simulink model "MPCtest1_real_44_double_lane_change"  (Simulink 8.7)
(part 2 of 4)

      | 6.247432626
      | 6.250432626
      | 6.253432626
      | 6.256432626
      | 6.259432626
      | 6.262432626
      | 6.265432626
      | 6.268432626
      | 6.271432626
      | 6.274432626
      | 6.277432626
      | 6.280432626
      | 6.283432626
      | 6.286432626
      | 6.289432626
      | 6.292432626
      | 6.295432626
      | 6.298432626
      | 6.301432626
      | 6.304432626
      | 6.307432626
      | 6.310432626
      | 6.313432626
      | 6.316432626
      | 6.319432626
      | ]*4
      | [0
      | 0
      | 0
      | 0
      | 0
      | 0
      | 0
      | 0
      | 0
      | 0
      | 0
      | 0
      | 0
      | 0
      | 0
      | 0
      | 0
      | 0
      | 0
      | 0
      | 0
      | 0
      | 0
      | 0
      | 0
      | 0
      | 0
      | 0
      | 0
      | 0
      | 0
      | 0
      | 0
      | 0
      | 0
      | 0
      | 0
      | 0
      | 0
      | 0
      | 0
      | 0
      | 0
      | 0
      | 0
      | 0
      | 0
      | 0
      | 0
      | 0
      | 0
      | 0
      | 0
      | 0
      | 0
      | 0
      | 0
      | 0
      | 0
      | 0
      | 0
      | 0
      | 0
      | 0
      | 0
      | 0
      | 0
      | 0
      | 0
      | 0
      | 0
      | 0
      | 0
      | 0
      | 0
      | 0
      | 0
      | 0
      | 0
      | 0
      | 0
      | 0
      | 0
      | 0
      | 0
      | 0
      | 0
      | 0
      | 0
      | 0
      | 0
      | 0
      | 0
      | 0
      | 0
      | 0
      | 0
      | 0
      | 0
      | 0
      | 0
      | 0
      | 0
      | 0
      | 0
      | 0
      | 0
      | 0
      | 0
      | 0
      | 0
      | 0
      | 0
      | 0
      | 0
      | 0
      | 0
      | 0
      | 0
      | 0
      | 0
      | 0
      | 0
      | 0
      | 0
      | 0
      | 0
      | 0
      | 0
      | 0
      | 0
      | 0
      | 0
      | 0
      | 0
      | 0
      | 0
      | 0
      | 0
      | 0
      | 0
      | 0
      | 0
      | 0
      | 0
      | 0
      | 0
      | 0
      | 0
      | 0
      | 0
      | 0
      | 0
      | 0
      | 0
      | 0
      | 0
      | 0
      | 0
      | 0
      | 0
      | 0
      | 0
      | 0
      | 0
      | 0
      | 0
      | 0
      | 0
      | 0
      | 0
      | 0
      | 0
      | 0
      | 0
      | 0
      | 0
      | 0
      | 0
      | 0
      | 0
      | 0
      | 0
      | 0
      | 0
      | 0
      | 0
      | 0
      | 0
      | 0
      | 0
      | 0
      | 0
      | 0
      | 0
      | 0
      | 0
      | 0
      | 0
      | 0
      | 0
      | 0
      | 0
      | 0
      | 0
      | 0
      | 0
      | 0
      | 0
      | 0
      | 0
      | 0
      | 0
      | 0
      | 0
      | 0
      | 0
      | 0
      | 0
      | 0
      | 0
      | 0
      | 0
      | 0
      | 0
      | 0
      | 0
      | 0
      | 0
      | 0
      | 0
      | 0
      | 0
      | 0
      | 0
      | 0
      | 0
      | 0
      | 0
      | 0
      | 0
      | 0
      | 0
      | 0
      | 0
      | 0
      | 0
      | 0
      | 0
      | 0
      | 0
      | 0
      | 0
      | 0
      | 0
      | 0
      | 0
      | 0
      | 0
      | 0
      | 0
      | 0
      | 0
      | 0
      | 0
      | 0
      | 0
      | 0
      | 0
      | 0
      | 0
      | 0
      | 0
      | 0
      | 0
      | 0
      | 0
      | 0
      | 0
      | 0
      | 0
      | 0
      | 0
      | 0
      | 0
      | 0
      | 0
      | 0
      | 0
      | 0
      | 0
      | 0
      | 0
      | 0
      | 0
      | 0
      | 0
      | 0
      | 0
      | 0
      | 0
      | 0
      | 0
      | 0
      | 0
      | 0
      | 0
      | 0
      | 0
      | 0
      | 0
      | 0
      | 0
      | 0
      | 0
      | 0
      | 0
      | 0
      | 0
      | 0
      | 0
      | 0
      | 0
      | 0
      | 0
      | 0
      | 0
      | 0
      | 0
      | 0
      | 0
      | 0
      | 0
      | 0
      | 0
      | 0
      | 0
      | 0
      | 0
      | 0
      | 0
      | 0
      | 0
      | 0
      | 0
      | 0
      | 0
      | 0
      | 0
      | 0
      | 0
      | 0
      | 0
      | 0
      | 0
      | 0
      | 0
      | 0
      | 0
      | 0
      | 0
      | 0
      | 0
      | 0
      | 0
      | 0
      | 0
      | 0
      | 0
      | 0
      | 0
      | 0
      | 0
      | 0
      | 0
      | 0
      | 0
      | 0
      | 0
      | 0
      | 0
      | 0
      | 0
      | 0
      | 0
      | 0
      | 0
      | 0
      | 0
      | 0
      | 0
      | 0
      | 0
      | 0
      | 0
      | 0
      | 0
      | 0
      | 0
      | 0
      | 0
      | 0
      | 0
      | 0
      | 0
      | 0
      | 0
      | 0
      | 0
      | 0
      | 0
      | 0
      | 0
      | 0
      | 0
      | 0
      | 0
      | 0
      | 0
      | 0
      | 0
      | 0
      | 0
      | 0
      | 0
      | 0
      | 0
      | 0
      | 0
      | 0
      | 0
      | 0
      | 0
      | 0
      | 0
      | 0
      | 0
      | 0
      | 0
      | 0
      | 0
      | 0
      | 0
      | 0
      | 0
      | 0
      | 0
      | 0
      | 0
      | 0
      | 0
      | 0
      | 0
      | 0
      | 0
      | 0
      | 0
      | 0
      | 0
      | 0
      | 0
      | 0
      | 0
      | 0
      | 0
      | 0
      | 0
      | 0
      | 0
      | 0
      | 0
      | 0
      | 0
      | 0
      | 0
      | 0
      | 0
      | 0
      | 0
      | 0
      | 0
      | 0
      | 0
      | 0
      | 0
      | 0
      | 0
      | 0
      | 0
      | 0
      | 0
      | 0
      | 0
      | 0
      | 0
      | 0
      | 0
      | 0
      | 0
      | 0
      | 0
      | 0
      | 0
      | 0
      | 0
      | 0
      | 0
      | 0
      | 0
      | 0
      | 0
      | 0
      | 0
      | 0
      | 0
      | 0
      | 0
      | 0
      | 0
      | 0
      | 0
      | 0
      | 0
      | 0
      | 0
      | 0
      | 0
      | 0
      | 0
      | 0
      | 0
      | 0
      | 0
      | 0
      | 0
      | 0
      | 0
      | 0
      | 0
      | 0
      | 0
      | 0
      | 0
      | 0
      | 0
      | 0
      | 0
      | 0
      | 0
      | 0
      | 0
      | 0
      | 0
      | 0
      | 0
      | 0
      | 0
      | 0
      | 0
      | 0
      | 0
      | 0
      | 0
      | 0
      | 0
      | 0
      | 0
      | 0
      | 0
      | 0
      | 0
      | 0
      | 0
      | 0
      | 0
      | 0
      | 0
      | 0
      | 0
      | 0
      | 0
      | 0
      | 0
      | 0
      | 0
      | 0
      | 0
      | 0
      | 0
      | 0
      | 0
      | 0
      | 0
      | 0
      | 0
      | 0
      | 0
      | 0
      | 0
      | 0
      | 0
      | 0
      | 0
      | 0
      | 0
      | 0
      | 0
      | 0
      | 0
      | 0
      | 0
      | 0
      | 0
      | 0
      | 0
      | 0
      | 0
      | 0
      | 0
      | 0
      | 0
      | 0
      | 0
      | 0
      | 0
      | 0
      | 0
      | 0
      | 0
      | 0
      | 0
      | 0
      | 0
      | 0.000684775
      | 0.001324361
      | 0.001984804
      | 0.002666103
      | 0.003368258
      | 0.004091268
      | 0.004835135
      | 0.005599859
      | 0.006385438
      | 0.007191873
      | 0.008019164
      | 0.008867312
      | 0.009736315
      | 0.010626175
      | 0.01153689
      | 0.012468462
      | 0.01342089
      | 0.01483377
      | 0.018465484
      | 0.024755628
      | 0.033704202
      | 0.045311203
      | 0.059576628
      | 0.076500472
      | 0.096082727
      | 0.118323378
      | 0.143222408
      | 0.170779791
      | 0.200995494
      | 0.233869472
      | 0.269401669
      | 0.307592013
      | 0.348440416
      | 0.391946773
      | 0.438110954
      | 0.486932806
      | 0.538412147
      | 0.592548768
      | 0.64934242
      | 0.708792823
      | 0.770899649
      | 0.835662532
      | 0.903081051
      | 0.973154735
      | 1.045883055
      | 1.12126542
      | 1.199301171
      | 1.27998958
      | 1.363329839
      | 1.449321062
      | 1.537962274
      | 1.629252408
      | 1.723190299
      | 1.819774678
      | 1.919004165
      | 2.020877268
      | 2.125392368
      | 2.23254772
      | 2.342341444
      | 2.454771518
      | 2.569835772
      | 2.687531878
      | 2.807857348
      | 2.930809523
      | 3.056385568
      | 3.184582462
      | 3.315396992
      | 3.448441077
      | 3.582173204
      | 3.716206863
      | 3.850540302
      | 3.985171745
      | 4.120099399
      | 4.255321449
      | 4.39083606
      | 4.526641376
      | 4.662735523
      | 4.799116606
      | 4.935782709
      | 5.072731897
      | 5.209962216
      | 5.347471689
      | 5.485258323
      | 5.623320104
      | 5.761654995
      | 5.900260946
      | 6.03913588
      | 6.178277707
      | 6.317684314
      | 6.457353569
      | 6.597283322
      | 6.737471404
      | 6.877915624
      | 7.018613777
      | 7.159563635
      | 7.300762953
      | 7.442209467
      | 7.583900896
      | 7.725834939
      | 7.868009277
      | 8.010421573
      | 8.153069473
      | 8.295950604
      | 8.439062575
      | 8.58240298
      | 8.725969392
      | 8.869759369
      | 9.013770452
      | 9.158000164
      | 9.302446012
      | 9.447105487
      | 9.591976061
      | 9.737055194
      | 9.882340325
      | 10.02782888
      | 10.17351827
      | 10.31940589
      | 10.46478504
      | 10.60684135
      | 10.74487929
      | 10.87890802
      | 11.00893664
      | 11.13497419
      | 11.25702959
      | 11.37511167
      | 11.48922913
      | 11.59939052
      | 11.70560423
      | 11.80787849
      | 11.90622133
      | 12.00064058
      | 12.09114386
      | 12.17773858
      | 12.26043189
      | 12.33923072
      | 12.41414171
      | 12.48517127
      | 12.55232551
      | 12.61561027
      | 12.67503108
      | 12.73059319
      | 12.78230154
      | 12.83016075
      | 12.87417512
      | 12.91434864
      | 12.95068495
      | 12.98318738
      | 13.0118589
      | 13.03670215
      | 13.05771942
      | 13.07491265
      | 13.08828345
      | 13.09783304
      | 13.10356233
      | 13.10547183
      | 13.10356174
      | 13.09783187
      | 13.08828168
      | 13.0749103
      | 13.05771647
      | 13.03669861
      | 13.01185477
      | 12.98318266
      | 12.95067964
      | 12.91434274
      | 12.87416863
      | 12.83015366
      | 12.78281531
      | 12.7342365
      | 12.68493774
      | 12.63491826
      | 12.58417732
      | 12.53271414
      | 12.48052795
      | 12.42761797
      | 12.37398342
      | 12.31962352
      | 12.26453747
      | 12.20872447
      | 12.15218373
      | 12.09491443
      | 12.03691577
      | 11.97818694
      | 11.91872712
      | 11.8585355
      | 11.79761124
      | 11.73595354
      | 11.67356155
      | 11.61043447
      | 11.54657144
      | 11.48197166
      | 11.41663428
      | 11.35055847
      | 11.2837434
      | 11.21618824
      | 11.14789216
      | 11.07885433
      | 11.00907391
      | 10.93855008
      | 10.867282
      | 10.79526886
      | 10.72250983
      | 10.64900409
      | 10.57475082
      | 10.49974921
      | 10.42399845
      | 10.34749774
      | 10.27024626
      | 10.19224323
      | 10.11348786
      | 10.03397935
      | 9.953716929
      | 9.872699826
      | 9.790927273
      | 9.708398512
      | 9.625112792
      | 9.54106937
      | 9.456179996
      | 9.370093566
      | 9.282721107
      | 9.194061124
      | 9.10411213
      | 9.012872647
      | 8.920341205
      | 8.826516347
      | 8.731396628
      | 8.634980618
      | 8.5372669
      | 8.438254076
      | 8.337940766
      | 8.23632561
      | 8.133407268
      | 8.029184426
      | 7.923655791
      | 7.8168201
      | 7.708676117
      | 7.599222632
      | 7.488458472
      | 7.376382494
      | 7.26299359
      | 7.148290688
      | 7.032272757
      | 6.914938803
      | 6.796287878
      | 6.676319074
      | 6.555031532
      | 6.432424439
      | 6.308497034
      | 6.183248606
      | 6.056678497
      | 5.928786109
      | 5.799570897
      | 5.66903238
      | 5.537170137
      | 5.403983812
      | 5.269473115
      | 5.133637825
      | 4.996477792
      | 4.857992938
      | 4.718183263
      | 4.57704884
      | 4.434589826
      | 4.290806458
      | 4.145699057
      | 3.999268032
      | 3.851513881
      | 3.702437191
      | 3.552764079
      | 3.405398667
      | 3.261070968
      | 3.119785508
      | 2.981546535
      | 2.846358023
      | 2.714223692
      | 2.58514701
      | 2.459131211
      | 2.336179303
      | 2.216294078
      | 2.099478122
      | 1.985733827
      | 1.875063399
      | 1.767468869
      | 1.662952101
      | 1.561514803
      | 1.463158534
      | 1.367884713
      | 1.27569463
      | 1.18658945
      | 1.100570225
      | 1.017637898
      | 0.937793314
      | 0.861037224
      | 0.787370295
      | 0.716793114
      | 0.649306195
      | 0.584909987
      | 0.523604877
      | 0.4653912
      | 0.410269237
      | 0.358239228
      | 0.309301372
      | 0.263455833
      | 0.220702745
      | 0.181042214
      | 0.144474324
      | 0.110999137
      | 0.080616703
      | 0.053327053
      | 0.029130212
      | 0.008026194
      | 0
      | 0
      | 0
      | 0
      | 0
      | 0
      | 0
      | 0
      | 0
      | 0
      | 0
      | 0
      | 0
      | 0
      | 0
      | 0
      | 0
      | 0
      | 0
      | 0
      | 0
      | 0
      | 0
      | 0
      | 0
      | 0
      | 0
      | 0
      | 0
      | 0
      | 0
      | 0
      | 0
      | 0
      | 0
      | 0
      | 0
      | 0
      | 0
      | 0
      | 0
      | 0
      | 0
      | 0
      | 0
      | 0
      | 0
      | 0
      | 0
      | 0
      | 0
      | 0
      | 0
      | 0
      | 0
      | 0
      | 0
      | 0
      | 0
      | 0
      | 0
      | 0
      | 0
      | 0
      | 0
      | 0
      | 0
      | 0
      | 0
      | 0
      | 0
      | 0
      | 0
      | 0
      | 0
      | 0
      | 0
      | 0
      | 0
      | 0
      | 0
      | 0
      | 0
      | 0
      | 0
      | 0
      | 0
      | 0
      | 0
      | 0
      | 0
      | 0
      | 0
      | 0
      | 0
      | 0
      | 0
      | 0
      | 0
      | 0
      | 0
      | 0
      | 0
      | 0
      | 0
      | 0
      | 0
      | 0
      | 0
      | 0
      | 0
      | 0
      | 0
      | 0
      | 0
      | 0
      | 0
      | 0
      | 0
      | 0
      | 0
      | 0
      | 0
      | 0
      | 0
      | 0
      | 0
      | 0
      | 0
      | 0
      | 0
      | 0
      | 0
      | 0
      | 0
      | 0
      | 0
      | 0
      | 0
      | 0
      | 0
      | 0
      | 0
      | 0
      | 0
      | 0
      | 0
      | 0
      | 0
      | 0
      | 0
      | 0
      | 0
      | 0
      | 0
      | 0
      | 0
      | 0
      | 0
      | 0
      | 0
      | 0
      | 0
      | 0
      | 0
      | 0
      | 0
      | 0
      | 0
      | 0
      | 0
      | 0
      | 0
      | 0
      | 0
      | 0
      | 0
      | 0
      | 0
      | 0
      | 0
      | 0
      | 0
      | 0
      | 0
      | 0
      | 0
      | 0
      | 0
      | 0
      | 0
      | 0
      | 0
      | 0
      | 0
      | 0
      | 0
      | 0
      | 0
      | 0
      | 0
      | 0
      | 0
      | 0
      | 0
      | 0
      | 0
      | 0
      | 0
      | 0
      | 0
      | 0
      | 0
      | 0
      | 0
      | 0
      | 0
      | 0
      | 0
      | 0
      | 0
      | 0
      | 0
      | 0
      | 0
      | 0
      | 0
      | 0
      | 0
      | 0
      | 0
      | 0
      | 0
      | 0
      | 0
      | 0
      | 0
      | 0
      | -0.004874691
      | -0.014693629
      | -0.02497131
      | -0.035707731
      | -0.046902892
      | -0.058556791
      | -0.070669428
      | -0.083240799
      | -0.096270904
      | -0.10975974
      | -0.123707304
      | -0.138113593
      | -0.152978604
      | -0.168302333
      | -0.184084776
      | -0.200325927
      | -0.217025783
      | -0.234184336
      | -0.251801581
      | -0.270432705
      | -0.292298463
      | -0.317954002
      | -0.347399255
      | -0.380634141
      | -0.417658552
      | -0.458472355
      | -0.503075382
      | -0.551467433
      | -0.603648259
      | -0.659617566
      | -0.719375
      | -0.782920146
      | -0.850252516
      | -0.921371543
      | -0.996276569
      | -1.074966841
      | -1.157441498
      | -1.243699558
      | -1.333739914
      | -1.427561316
      | -1.525162364
      | -1.626541494
      | -1.731696965
      | -1.840626846
      | -1.953329005
      | -2.069801091
      | -2.190040522
      | -2.314044468
      | -2.44180984
      | -2.573333271
      | -2.708611097
      | -2.847639349
      | -2.990413727
      | -3.136929589
      | -3.287181929
      | -3.441165362
      | -3.598874106
      | -3.76030196
      | -3.925442288
      | -4.094287998
      | -4.266831525
      | -4.443064808
      | -4.622979273
      | -4.806565811
      | -4.993814758
      | -5.184715876
      | -5.37925833
      | -5.577430671
      | -5.77922081
      | -5.983683309
      | -6.187078976
      | -6.388473667
      | -6.587866874
      | -6.785258334
      | -6.980648017
      | -7.174036124
      | -7.365423077
      | -7.554809509
      | -7.742196265
      | -7.927584385
      | -8.110975105
      | -8.292369844
      | -8.471770203
      | -8.649177951
      | -8.824595025
      | -8.998023519
      | -9.169465681
      | -9.338923903
      | -9.506400716
      | -9.671898783
      | -9.835420897
      | -9.996969969
      | -10.15654902
      | -10.3141612
      | -10.46980973
      | -10.62349795
      | -10.77522929
      | -10.92500726
      | -11.07283546
      | -11.21871755
      | -11.36265727
      | -11.50465843
      | -11.6447249
      | -11.78286059
      | -11.91906948
      | -12.05335559
      | -12.18572296
      | -12.31617571
      | -12.44471796
      | -12.57135386
      | -12.6960876
      | -12.81892339
      | -12.93986543
      | -13.05891796
      | -13.17608522
      | -13.29137145
      | -13.4047809
      | -13.51631782
      | -13.62598644
      | -13.733366
      | -13.83676348
      | -13.93576441
      | -14.03037933
      | -14.12061844
      | -14.20649156
      | -14.28800814
      | -14.3651772
      | -14.43800738
      | -14.50650689
      | -14.57068349
      | -14.63054452
      | -14.68609686
      | -14.73734695
      | -14.78430073
      | -14.82696369
      | -14.86534084
      | -14.8994367
      | -14.9292553
      | -14.95480018
      | -14.97607437
      | -14.9930804
      | -15.00582032
      | -15.01429564
      | -15.01850737
      | -15.01845602
      | -15.01414159
      | -15.00556355
      | -14.99272089
      | -14.97561206
      | -14.95423502
      | -14.92858723
      | -14.89866563
      | -14.86446668
      | -14.82598634
      | -14.78322008
      | -14.73616287
      | -14.68480921
      | -14.62915315
      | -14.56918824
      | -14.50490759
      | -14.43630386
      | -14.36336925
      | -14.28609556
      | -14.20447414
      | -14.11849595
      | -14.02815155
      | -13.93343109
      | -13.83432438
      | -13.73082086
      | -13.62333707
      | -13.51357441
      | -13.40195577
      | -13.28847693
      | -13.17313368
      | -13.05592182
      | -12.93683713
      | -12.81587542
      | -12.69303249
      | -12.56830415
      | -12.44168625
      | -12.31317465
      | -12.18276521
      | -12.05045386
      | -11.91623653
      | -11.78010922
      | -11.64206793
      | -11.50210874
      | -11.36022776
      | -11.21642118
      | -11.07068523
      | -10.9230162
      | -10.77341046
      | -10.62186447
      | -10.46837475
      | -10.31293791
      | -10.15555065
      | -9.996209768
      | -9.834912172
      | -9.67165487
      | -9.506434983
      | -9.339249755
      | -9.170096554
      | -8.998972882
      | -8.825876375
      | -8.650804816
      | -8.473756139
      | -8.294728432
      | -8.11371995
      | -7.930729116
      | -7.74575453
      | -7.558794976
      | -7.36984943
      | -7.178917063
      | -6.985997253
      | -6.791089588
      | -6.594193874
      | -6.395310146
      | -6.194438669
      | -5.991579951
      | -5.787657205
      | -5.58636586
      | -5.388640283
      | -5.194492424
      | -5.003933604
      | -4.816974542
      | -4.633625375
      | -4.453895672
      | -4.277794461
      | -4.105330244
      | -3.936511016
      | -3.771344291
      | -3.60983711
      | -3.451996072
      | -3.297827344
      | -3.147336681
      | -3.000529449
      | -2.857410636
      | -2.717984874
      | -2.582256455
      | -2.450229347
      | -2.321907213
      | -2.197293424
      | -2.076391075
      | -1.959203003
      | -1.845731801
      | -1.73597983
      | -1.629949237
      | -1.527641965
      | -1.42905977
      | -1.334204229
      | -1.243076759
      | -1.155678622
      | -1.072010941
      | -0.992074711
      | -0.915870806
      | -0.843399993
      | -0.774662941
      | -0.709660228
      | -0.648392351
      | -0.590859735
      | -0.537062741
      | -0.48700167
      | -0.440676777
      | -0.398088267
      | -0.359236311
      | -0.324121046
      | -0.29274258
      | -0.265100999
      | -0.241196368
      | -0.220513931
      | -0.200994493
      | -0.182123257
      | -0.163900232
      | -0.146325425
      | -0.129398844
      | -0.113120493
      | -0.097490378
      | -0.082508503
      | -0.068174871
      | -0.054489486
      | -0.041452351
      | -0.029063467
      | -0.017322835
      | -0.006230459
      | 0.004213663
      | 0.014009528
      | 0.023157137
      | 0.031656489
      | 0.039507584
      | 0.046710423
      | 0.053265004
      | 0.059171329
      | 0.064429398
      | 0.069039211
      | 0.073000768
      | 0.07631407
      | 0.078979117
      | 0.080995909
      | 0.082364446
      | 0.083084729
      | 0.083156757
      | 0.082580531
      | 0.08135605
      | 0.079483315
      | 0.076962325
      | 0.07379308
      | 0.069975579
      | 0.065509823
      | 0.060395811
      | 0.054773598
      | 0.049203405
      | 0.043825286
      | 0.038639242
      | 0.033645273
      | 0.02884338
      | 0.024233562
      | 0.019815819
      | 0.015590152
      | 0.01155656
      | 0.007715044
      | 0.004065604
      | 0.00060824
      | 0
      | 0
      | 0
      | 0
      | 0
      | 0
      | 0
      | 0
      | 0
      | 0
      | 0
      | 0
      | 0
      | 0
      | 0
      | 0
      | 0
      | 0
      | 0
      | 0
      | 0
      | 0
      | 0
      | 0
      | 0
      | 0
      | 0
      | 0
      | 0
      | 0
      | 0
      | 0
      | 0
      | 0
      | 0
      | 0
      | 0
      | 0
      | 0
      | 0
      | 0
      | 0
      | 0
      | 0
      | 0
      | 0
      | 0
      | 0
      | 0
      | 0
      | 0
      | 0
      | 0
      | 0
      | 0
      | 0
      | 0
      | 0
      | 0
      | 0
      | 0
      | 0
      | 0
      | 0
      | 0
      | 0
      | 0
      | 0
      | 0
      | 0
      | 0
      | 0
      | 0
      | 0
      | 0
      | 0
      | 0
      | 0
      | 0
      | 0
      | 0
      | 0
      | 0
      | 0
      | 0
      | 0
      | 0
      | 0
      | 0
      | 0
      | 0
      | 0
      | 0
      | 0
      | 0
      | 0
      | 0
      | 0
      | 0
      | 0
      | 0
      | 0
      | 0
      | 0
      | 0
      | 0
      | 0
      | 0
      | 0
      | 0
      | 0
      | 0
      | 0
      | 0
      | 0
      | 0
      | 0
      | 0
      | 0
      | 0
      | 0
      | 0
      | 0
      | 0
      | 0
      | 0
      | 0
      | 0
      | 0
      | 0
      | 0
      | 0
      | 0
      | 0
      | 0
      | 0
      | 0
      | 0
      | 0
      | 0
      | 0
      | 0
      | 0
      | 0
      | 0
      | 0
      | 0
      | 0
      | 0
      | 0
      | 0
      | 0
      | 0
      | 0
      | 0
      | 0
      | 0
      | 0
      | 0
      | 0
      | 0
      | 0
      | 0
      | 0
      | 0
      | 0
      | 0
      | 0
      | 0
      | 0
      | 0
      | 0
      | 0
      | 0
      | 0
      | 0
      | 0
      | 0
      | 0
      | 0
      | 0
      | 0
      | 0
      | 0
      | 0
      | 0
      | 0
      | 0
      | 0
      | 0
      | 0
      | 0
      | 0
      | 0
      | 0
      | 0
      | 0
      | 0
      | 0
      | 0
      | 0
      | 0
      | 0
      | 0
      | 0
      | 0
      | 0
      | 0
      | 0
      | 0
      | 0
      | 0
      | 0
      | 0
      | 0
      | 0
      | 0
      | 0
      | 0
      | 0
      | 0
      | 0
      | 0
      | 0
      | 0
      | 0
      | 0
      | 0
      | 0
      | 0
      | 0
      | 0
      | 0
      | 0
      | 0
      | 0
      | 0
      | 0
      | 0
      | 0
      | 0
      | 0
      | 0
      | 0
      | 0
      | 0
      | 0
      | 0
      | 0
      | 0
      | 0
      | 0
      | 0
      | 0
      | 0
      | 0
      | 0
      | 0
      | 0
      | 0
      | 0
      | 0
      | 0
      | 0
      | 0
      | 0
      | 0
      | 0
      | 0
      | 0
      | 0
      | 0
      | 0
      | 0
      | 0
      | 0
      | 0
      | 0
      | 0
      | 0
      | 0
      | 0
      | 0
      | 0
      | 0
      | 0
      | 0
      | 0
      | 0
      | 0
      | 0
      | 0
      | 0
      | 0
      | 0
      | 0
      | 0
      | 0
      | 0
      | 0
      | 0
      | 0
      | 0
      | 0
      | 0
      | 0
      | 0
      | 0
      | 0
      | 0
      | 0
      | 0
      | 0
      | 0
      | 0
      | 0
      | 0
      | 0
      | 0
      | 0
      | 0
      | 0
      | 0
      | 0
      | 0
      | 0
      | 0
      | 0
      | 0
      | 0
      | 0
      | 0
      | 0
      | 0
      | 0
      | 0
      | 0
      | 0
      | 0
      | 0
      | 0
      | 0
      | 0
      | 0
      | 0
      | 0
      | 0
      | 0
      | 0
      | 0
      | 0
      | 0
      | 0
      | 0
      | 0
      | 0
      | 0
      | 0
      | 0
      | 0
      | 0
      | 0
      | 0
      | 0
      | 0
      | 0
      | 0
      | 0
      | 0
      | 0
      | 0
      | 0
      | 0
      | 0
      | 0
      | 0
      | 0
      | 0
      | 0
      | 0
      | 0
      | 0
      | 0
      | 0
      | 0
      | 0
      | 0
      | 0
      | 0
      | 0
      | 0
      | 0
      | 0
      | 0
      | 0
      | 0
      | 0
      | 0
      | 0
      | 0
      | 0
      | 0
      | 0
      | 0
      | 0
      | 0
      | 0
      | 0
      | 0
      | 0
      | 0
      | 0
      | 0
      | 0
      | 0
      | 0
      | 0
      | 0
      | 0
      | 0
      | 0
      | 0
      | 0
      | 0
      | 0
      | 0
      | 0
      | 0
      | 0
      | 0
      | 0
      | 0
      | 0
      | 0
      | 0
      | 0
      | 0
      | 0
      | 0
      | 0
      | 0
      | 0
      | 0
      | 0
      | 0
      | 0
      | 0
      | 0
      | 0
      | 0
      | 0
      | 0
      | 0
      | 0
      | 0
      | 0
      | 0
      | 0
      | 0
      | 0
      | 0
      | 0
      | 0
      | 0
      | 0
      | 0
      | 0
      | 0
      | 0
      | 0
      | 0
      | 0
      | 0
      | 0
      | 0
      | 0
      | 0
      | 0
      | 0
      | 0
      | 0
      | 0
      | 0
      | 0
      | 0
      | 0
      | 0
      | 0
      | 0
      | 0
      | 0
      | 0
      | 0
      | 0
      | 0
      | 0
      | 0
      | 0
      | 0
      | 0
      | 0
      | 0
      | 0
      | 0
      | 0
      | 0
      | 0
      | 0
      | 0
      | 0
      | 0
      | 0
      | 0
      | 0
      | 0
      | 0
      | 0
      | 0
      | 0
      | 0
      | 0
      | 0
      | 0
      | 0
      | 0
      | 0
      | 0
      | 0
      | 0
      | 0
      | 0
      | 0
      | 0
      | 0
      | 0
      | 0
      | 0
      | 0
      | 0
      | 0
      | 0
      | 0
      | 0
      | 0
      | 0
      | 0
      | 0
      | 0
      | 0
      | 0
      | 0
      | 0
      | 0
      | 0
      | 0
      | 0
      | 0
      | 0
      | 0
      | 0
      | 0
      | 0
      | 0
      | 0
      | 0
      | 0
      | 0
      | 0
      | 0
      | 0
      | 0
      | 0
      | 0
      | 0
      | 0
      | 0
      | 0
      | 0
      | 0
      | 0
      | 0
      | 0
      | 0
      | 0
      | 0
      | 0
      | 0
      | 0
      | 0
      | 0
      | 0
      | 0
      | 0
      | 0
      | 0
      | 0
      | 0
      | 0
      | ]
  15epoch : Subsystem  mask{pi_input_1_delayed_1=[0;0;0;0], pi_input_1_delayed_2=[0;0;0;0], pi_input_1_delayed_3=[0;0;0;0]}
      mask prompts: pi_input_1_delayed_1 "Preprocessed initial input 1 state at timestep 0."; pi_input_1_delayed_2 "Preprocessed initial input 1 state at timestep -1."; pi_input_1_delayed_3 "Preprocessed initial input 1 state at timestep -2."
      mask help: Time Delay Neural Network
      mask Display: e = 0.06;c1 = [120 150 230]/255;c2 = ([120 150 230]+0)/383;c3 = ([120 150 230]+128)/383;patch([0 1 1 0],[0 0 1 1],c1);patch([0 1 1 1-e 1-e 0+e],[0 0 1 1-e 0+e 0+e],c2);patch([0 0 1 1-e 0+e 0+e],[0 1 1 1-e 1-e 0+e],c3);plot([0 1 1 0 0],[0 0 1 1 0]);fprintf('NNET');port_label('input',1,' x');port_label('output',1,'y ');
  15epoch_2 用的0.2s_0.02_2的数据 : Subsystem  mask{pi_input_1_delayed_1=[0;0;0;0], pi_input_1_delayed_2=[0;0;0;0], pi_input_1_delayed_3=[0;0;0;0]}
      mask prompts: pi_input_1_delayed_1 "Preprocessed initial input 1 state at timestep 0."; pi_input_1_delayed_2 "Preprocessed initial input 1 state at timestep -1."; pi_input_1_delayed_3 "Preprocessed initial input 1 state at timestep -2."
      mask help: Time Delay Neural Network
      mask Display: e = 0.06;c1 = [120 150 230]/255;c2 = ([120 150 230]+0)/383;c3 = ([120 150 230]+128)/383;patch([0 1 1 0],[0 0 1 1],c1);patch([0 1 1 1-e 1-e 0+e],[0 0 1 1-e 0+e 0+e],c2);patch([0 0 1 1-e 0+e 0+e],[0 1 1 1-e 1-e 0+e],c3);plot([0 1 1 0 0],[0 0 1 1 0]);fprintf('NNET');port_label('input',1,' x');port_label('output',1,'y ');
  60:360训练的 : Subsystem  mask{pi_input_1_delayed_1=[0;0;0;0], pi_input_1_delayed_2=[0;0;0;0], pi_input_1_delayed_3=[0;0;0;0]}
      mask prompts: pi_input_1_delayed_1 "Preprocessed initial input 1 state at timestep 0."; pi_input_1_delayed_2 "Preprocessed initial input 1 state at timestep -1."; pi_input_1_delayed_3 "Preprocessed initial input 1 state at timestep -2."
      mask help: Time Delay Neural Network
      mask Display: e = 0.06;c1 = [120 150 230]/255;c2 = ([120 150 230]+0)/383;c3 = ([120 150 230]+128)/383;patch([0 1 1 0],[0 0 1 1],c1);patch([0 1 1 1-e 1-e 0+e],[0 0 1 1-e 0+e 0+e],c2);patch([0 0 1 1-e 0+e 0+e],[0 1 1 1-e 1-e 0+e],c3);plot([0 1 1 0 0],[0 0 1 1 0]);fprintf('NNET');port_label('input',1,' x');port_label('output',1,'y ');
  Abs : Abs
  Add : Sum  Inputs=+-
  Add1 : Sum  Inputs=+-
  CarSim S-Function : Solver_SF/CarSim S-Function  Priority=1  VehicleCode=i_i  SIMFILE=simfile.sim
  Clock1 : Clock
  Clock2 : Clock
  Constant2 : Constant  Value=0
  Demux : Demux  Outputs=9
  Demux1 : Demux  Outputs=2
  Gain : Gain  Gain=3.6
  Gain1 : Gain  Gain=1/3.6
  Gain10 : Gain
  Gain11 : Gain  Gain=1/0.05
  Gain2 : Gain  Gain=3.14/180
  Gain3 : Gain  Gain=0.4
  Gain4 : Gain  Gain=1/0.05
  Gain5 : Gain  Gain=180/3.14
  Gain6 : Gain  Gain=16.28
  Gain7 : Gain  Gain=2/3
  Mux1 : Mux  Inputs=3
  Mux3 : Mux  Inputs=6
  Mux4 : Mux  Inputs=2
  Mux5 : Mux  Inputs=3
  "PID " : simulink/Continuous/PID Controller  Controller=PID  TimeDomain=Discrete-time  SampleTime=0.05  IntegratorMethod=Forward Euler  FilterMethod=Forward Euler  Form=Parallel  UseFilter=off  ControllerParametersSource=internal  P=1  I=0  D=-0.01  N=10  InitialConditionSource=internal  InitialConditionForIntegrator=0  InitialConditionForFilter=0  ExternalReset=none  LimitOutput=off  UpperSaturationLimit=inf  LowerSaturationLimit=-inf  LinearizeAsGain=off  AntiWindupMode=none  Kb=1  TrackingMode=off  Kt=1  PParamMin=[]  PParamMax=[]  IParamMin=[]  IParamMax=[]  DParamMin=[]  DParamMax=[]  NParamMin=[]  NParamMax=[]  KbParamMin=[]  KbParamMax=[]  KtParamMin=[]  KtParamMax=[]  POutMin=[]  POutMax=[]  IOutMin=[]  IOutMax=[]  DOutMin=[]  DOutMax=[]  NOutMin=[]  NOutMax=[]  KbOutMin=[]  KbOutMax=[]  KtOutMin=[]  KtOutMax=[]  IntegratorOutMin=[]  IntegratorOutMax=[]  FilterOutMin=[]  FilterOutMax=[]  SumOutMin=[]  SumOutMax=[]  SumI1OutMin=[]  SumI1OutMax=[]  SumI2OutMin=[]  SumI2OutMax=[]  SumI3OutMin=[]  SumI3OutMax=[]  SumDOutMin=[]  SumDOutMax=[]  SaturationOutMin=[]  SaturationOutMax=[]  IntegratorContinuousStateAttributes=''  IntegratorStateMustResolveToSignalObject=off  IntegratorRTWStateStorageClass=Auto  FilterContinuousStateAttributes=''  FilterStateMustResolveToSignalObject=off  FilterRTWStateStorageClass=Auto  DifferentiatorICPrevScaledInput=0  DifferentiatorOutMin=[]  DifferentiatorOutMax=[]
  PID 1 : simulink/Continuous/PID Controller  Controller=PID  TimeDomain=Discrete-time  SampleTime=0.05  IntegratorMethod=Forward Euler  FilterMethod=Forward Euler  Form=Parallel  UseFilter=off  ControllerParametersSource=internal  P=1  I=-2  D=0.02  N=10  InitialConditionSource=internal  InitialConditionForIntegrator=0  InitialConditionForFilter=0  ExternalReset=either  LimitOutput=off  UpperSaturationLimit=inf  LowerSaturationLimit=-inf  LinearizeAsGain=off  AntiWindupMode=none  Kb=1  TrackingMode=off  Kt=1  PParamMin=[]  PParamMax=[]  IParamMin=[]  IParamMax=[]  DParamMin=[]  DParamMax=[]  NParamMin=[]  NParamMax=[]  KbParamMin=[]  KbParamMax=[]  KtParamMin=[]  KtParamMax=[]  POutMin=[]  POutMax=[]  IOutMin=[]  IOutMax=[]  DOutMin=[]  DOutMax=[]  NOutMin=[]  NOutMax=[]  KbOutMin=[]  KbOutMax=[]  KtOutMin=[]  KtOutMax=[]  IntegratorOutMin=[]  IntegratorOutMax=[]  FilterOutMin=[]  FilterOutMax=[]  SumOutMin=[]  SumOutMax=[]  SumI1OutMin=[]  SumI1OutMax=[]  SumI2OutMin=[]  SumI2OutMax=[]  SumI3OutMin=[]  SumI3OutMax=[]  SumDOutMin=[]  SumDOutMax=[]  SaturationOutMin=[]  SaturationOutMax=[]  IntegratorContinuousStateAttributes=''  IntegratorStateMustResolveToSignalObject=off  IntegratorRTWStateStorageClass=Auto  FilterContinuousStateAttributes=''  FilterStateMustResolveToSignalObject=off  FilterRTWStateStorageClass=Auto  DifferentiatorICPrevScaledInput=0  DifferentiatorOutMin=[]  DifferentiatorOutMax=[]
  PID弯道 : Scope  NumInputPorts=2
  PID直道 : Scope  NumInputPorts=2
  Random Number : RandomNumber  Variance=0.0005  SampleTime=0.1
  S-Function : S-Function  FunctionName=MY_MPCController3_double_lane_change  SFunctionDeploymentMode=off  EnableBusSupport=off
  Saturation1 : Saturate  UpperLimit=0.08  LowerLimit=-0.08
  Subtract{1,7..9} (4 alike) : Sum  Inputs=+-
  Subtract11 : Sum
  Subtract2 : Sum
  Subtract3 : Sum
  Switch1 : Switch  Criteria=u2 > Threshold  Threshold=1
  Switch3 : Switch  Criteria=u2 > Threshold  Threshold=7
  To Workspace : ToWorkspace  VariableName=x_real  SaveFormat=Timeseries  SampleTime=-1
  To Workspace1 : ToWorkspace  VariableName=y_real  SaveFormat=Timeseries  SampleTime=-1
  To Workspace2 : ToWorkspace  VariableName=x_predict  SaveFormat=Timeseries  SampleTime=-1
  To Workspace3 : ToWorkspace  VariableName=y_predict  SaveFormat=Timeseries  SampleTime=-1
  To Workspace4 : ToWorkspace  VariableName=v_predict  SaveFormat=Timeseries  SampleTime=-1
  To Workspace5 : ToWorkspace  VariableName=v_real  SaveFormat=Timeseries  SampleTime=-1
  To Workspace6 : ToWorkspace  VariableName=steer_torque  SaveFormat=Timeseries  SampleTime=-1
  To Workspace7 : ToWorkspace  VariableName=Ay  SaveFormat=Timeseries  SampleTime=-1
  To Workspace8 : ToWorkspace  VariableName=Vy  SaveFormat=Timeseries  SampleTime=-1
  Unit Delay : UnitDelay  SampleTime=-1
  Unit Delay1 : UnitDelay  SampleTime=-1
  XY Graph : simulink/Sinks/XY Graph  xmin=0  xmax=200  ymin=-2  ymax=5  st=-1
  XY Graph1 : simulink/Sinks/XY Graph  xmin=0  xmax=200  ymin=-2  ymax=5  st=-1
  X误差 : Scope
  YAW偏差 : Scope
  Y误差 : Scope
  Zero-Order Hold{,1..11} (12 alike) : ZeroOrderHold  SampleTime=0.05
  omega : ToWorkspace  VariableName=omega  SaveFormat=Timeseries  SampleTime=-1
  real车速km/h : Scope
  yaw : Scope
  yaw变化率 : Scope
  仿真yaw : Scope
  前轮角度rad : Scope
  前轮角速度rad/s : Scope
  前轮转角 ° : Scope  NumInputPorts=2
  前轮转角控制量rad : ToWorkspace  VariableName=delta_predict  SaveFormat=Timeseries  SampleTime=-1
  前轮转角控制量rad' : Scope
  前轮转角控制量rad1 : ToWorkspace  VariableName=delta_predict2  SaveFormat=Timeseries  SampleTime=-1
  实际前轮转角rad : ToWorkspace  VariableName=delta_real  SaveFormat=Timeseries  SampleTime=-1
  实际前轮转角rad' : Scope
  延迟时间 : Gain  Gain=0.2
  方向盘控制量 rad : Scope
  方向盘转矩 : Scope
  方向盘随机误差 rad : Scope
  横向加速度 : Scope
  横向速度 : Scope
  没有延时 °1 : Scope  NumInputPorts=2
  补偿 : Scope
  补偿后/实际值对比 : Scope  NumInputPorts=2
  补偿后/控制量 : Scope  NumInputPorts=2
  车速 : Constant  Value=30
  限制前/后 : Scope  NumInputPorts=2
  除去了predict-real重新训练 用的0.2s_0.02_2的数据 : Subsystem  mask{pi_input_1_delayed_1=[0;0;0], pi_input_1_delayed_2=[0;0;0], pi_input_1_delayed_3=[0;0;0]}
      mask prompts: pi_input_1_delayed_1 "Preprocessed initial input 1 state at timestep 0."; pi_input_1_delayed_2 "Preprocessed initial input 1 state at timestep -1."; pi_input_1_delayed_3 "Preprocessed initial input 1 state at timestep -2."
      mask help: Time Delay Neural Network
      mask Display: e = 0.06;c1 = [120 150 230]/255;c2 = ([120 150 230]+0)/383;c3 = ([120 150 230]+128)/383;patch([0 1 1 0],[0 0 1 1],c1);patch([0 1 1 1-e 1-e 0+e],[0 0 1 1-e 0+e 0+e],c2);patch([0 0 1 1-e 0+e 0+e],[0 1 1 1-e 1-e 0+e],c3);plot([0 1 1 0 0],[0 0 1 1 0]);fprintf('NNET');port_label('input',1,' x');port_label('output',1,'y ');
  wires:
  CarSim S-Function/1 -> Demux/1
  Demux/3 -> 仿真yaw/1, Subtract9/2, Mux1/3
  Demux/2 -> Zero-Order Hold8/1, Subtract8/2, XY Graph1/2, Mux1/2
  S-Function/1 -> Demux1/1
  Unit Delay/1 -> Mux3/1
  Demux1/1 -> Gain/1
  Demux1/2 -> Subtract3/2, 补偿后/实际值对比/1, 0.05s1/1, 前轮转角控制量rad'/1, 前轮转角控制量rad/1, 前轮角度rad/1, 0.05s2/1, Add/1, Mux5/1, Subtract1/1  "现在期望量"
  Zero-Order Hold/1 -> 1-D Lookup x/1, 1-D Lookup y/1, 1-D Lookup yaw/1
  1-D Lookup x/1 -> To Workspace2/1, XY Graph/1, Subtract7/1, Mux3/2  "x"
  1-D Lookup y/1 -> XY Graph/2, To Workspace3/1, Subtract8/1, Mux3/3  "y"
  Mux1/1 -> Unit Delay/1
  Clock1/1 -> Zero-Order Hold/1
  Mux3/1 -> S-Function/1
  1-D Lookup yaw/1 -> Subtract9/1, yaw/1, Add1/1, 0.05s3/1, Mux3/4  "yaw"
  Demux/1 -> Mux1/1, XY Graph1/1, Zero-Order Hold9/1, Subtract7/2
  Mux4/1 -> CarSim S-Function/1
  车速/1 -> To Workspace4/1, Gain1/1
  Demux/6 -> Zero-Order Hold3/1, 前轮转角 °/1  "1"
  Random Number/1 -> 方向盘随机误差 rad/1
  Subtract2/1 -> 方向盘控制量 rad/1, Gain5/1
  Gain6/1 -> Subtract2/1
  Demux/4 -> Unit Delay1/1, Zero-Order Hold2/1  "v(km/h)"
  Unit Delay1/1 -> real车速km/h/1, Mux3/5
  Demux/7 -> Zero-Order Hold1/1
  Zero-Order Hold1/1 -> Mux5/2, 方向盘转矩/1, To Workspace6/1
  Zero-Order Hold3/1 -> 前轮转角 °/2, Gain2/1  "2"
  Zero-Order Hold2/1 -> To Workspace5/1
  Mux5/1 -> 除去了predict-real重新训练 用的0.2s_0.02_2的数据/1(x)
  Gain2/1 -> 实际前轮转角rad'/1, Subtract11/1, Subtract1/2, 实际前轮转角rad/1  "实际前轮转角rad"
  Gain1/1 -> Mux3/6
  Subtract7/1 -> Zero-Order Hold4/1
  Subtract8/1 -> Zero-Order Hold5/1
  Zero-Order Hold4/1 -> X误差/1
  Zero-Order Hold5/1 -> Y误差/1
  Subtract9/1 -> Zero-Order Hold6/1
  Zero-Order Hold6/1 -> YAW偏差/1
  Gain/1 -> Mux4/1
  Gain11/1 -> 前轮角速度rad/s/1, Mux5/3, omega/1, 延迟时间/1  "前轮角速度rad/s"
  0.05s2/1 -> Add/2
  Gain10/1 -> Gain11/1
  Add/1 -> Gain10/1
  0.15s/1 -> Subtract11/2  "0.3秒前控制+补偿"
  Subtract11/1 -> 补偿后/控制量/2
  Subtract3/1 -> Gain6/1, 没有延时 °1/2, Zero-Order Hold7/1, 0.2s1/1  "补偿后的控制量"
  Saturation1/1 -> Switch3/1, 限制前/后/2
  Clock2/1 -> Switch3/2
  Switch3/1 -> Subtract3/1
  Constant2/1 -> Switch3/3
  延迟时间/1 -> 0.15s/1, 补偿/1
  0.05s1/1 -> 补偿后/控制量/1
  Gain5/1 -> 0.2s/1
  0.2s/1 -> Mux4/2
  0.2s1/1 -> 补偿后/实际值对比/2  "0.2s前补偿后的控制量"
  Zero-Order Hold7/1 -> 前轮转角控制量rad1/1, 没有延时 °1/1
  "PID "/1 -> Switch1/1, PID弯道/2  "弯道"
  0.05s3/1 -> Add1/2
  Add1/1 -> Gain4/1
  Gain4/1 -> yaw变化率/1, Abs/1
  Abs/1 -> Switch1/2
  除去了predict-real重新训练 用的0.2s_0.02_2的数据/1(y) -> Gain7/1, Gain3/1
  PID 1/1 -> PID直道/2, Switch1/3  "直道"
  Switch1/1 -> 限制前/后/1, Saturation1/1
  Gain7/1 -> PID弯道/1, "PID "/1
  Gain3/1 -> PID 1/2, PID 1/1, PID直道/1
  Zero-Order Hold8/1 -> To Workspace1/1
  Zero-Order Hold9/1 -> To Workspace/1
  Demux/8 -> Zero-Order Hold10/1
  Zero-Order Hold10/1 -> 横向加速度/1, To Workspace7/1
  Demux/9 -> Zero-Order Hold11/1
  Zero-Order Hold11/1 -> 横向速度/1, To Workspace8/1
